simulink model "sampleModel1692"  (R2023a)
settings: Solver=VariableStepAuto  StartTime=0.0  StopTime=10.0  RelTol=1e-3
libraries: hdlsllib x6, simulink x2
settings Model: Creator=user1  LastModifiedBy=user1

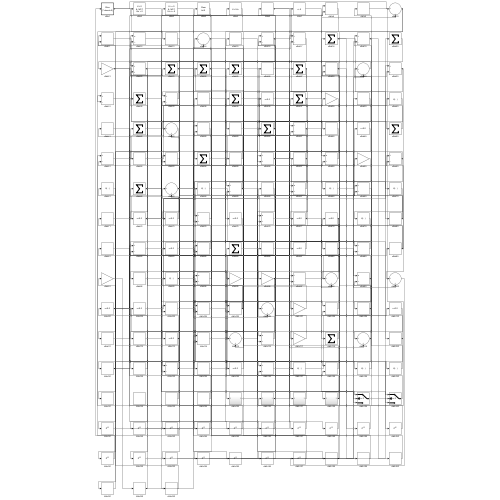
[thumbnail: Simulink's stored preview of the top-level diagram]
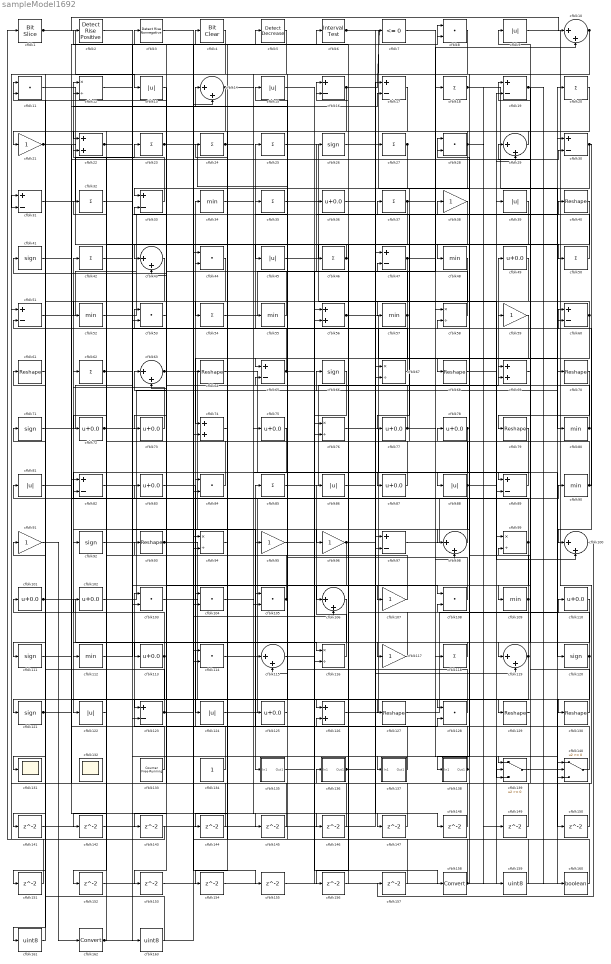
== system sampleModel1692 ==
  cfblk1 : hdlsllib/Logic and Bit Operations/Bit Slice  lidx=7  ridx=0
  cfblk{10,14,29,43,63,98,100,106,115,119} (10 alike) : Sum  Inputs=|++
  cfblk{36,49,72..73,75,77..78,83,87,101..102,110,113,125} (14 alike) : Bias  Bias=0.0  SaturateOnIntegerOverflow=off
  cfblk{8,11,28,44,53,84,103..105,108,114,128} (12 alike) : DotProduct  OutDataTypeStr=Inherit: Inherit via internal rule
  cfblk{21,38,59,91,95..96,107,117} (8 alike) : Gain
  cfblk{34,48,52,55,57,80,90,109,112} (9 alike) : MinMax
  cfblk{26,41,66,71,92,111,120..121} (8 alike) : Signum
  cfblk{12,58,67,76,94,99,116} (7 alike) : Product  Inputs=*/  RndMeth=Zero  SaturateOnIntegerOverflow=on
  cfblk{18,20,23..25,27,32,35,37,42,46,50,54,62,85,118} (16 alike) : Sum  Inputs=+
  cfblk{9,13,15,39,45,81,86,88,122,124} (10 alike) : Abs  SaturateOnIntegerOverflow=off
  cfblk{16..17,19,30..31,33,47,51,60,65,82,89,97,123} (14 alike) : Sum  Inputs=+-
  cfblk{22,56,69,74,126} (5 alike) : Sum
  cfblk{40,61,64,68,70,79,93,127,129..130} (10 alike) : Reshape
  cfblk131 : Scope
  cfblk132 : Scope
      settings: Floating=on
  cfblk133 : hdlsllib/Sources/Counter Free-Running  NumBits=16  tsamp=-1
  cfblk134 : Constant  SampleTime=-1
  cfblk135 : Subsystem
      settings: LibrarySourceBlock=|
      | hdlsllib/Ports &
      | Subsystems/Subsystem
  cfblk136 : Subsystem
      settings: LibrarySourceBlock=|
      | hdlsllib/Ports &
      | Subsystems/Subsystem
  cfblk137 : Subsystem
      settings: LibrarySourceBlock=|
      | hdlsllib/Ports &
      | Subsystems/Subsystem
  cfblk138 : Subsystem
      settings: LibrarySourceBlock=|
      | hdlsllib/Ports &
      | Subsystems/Subsystem
  cfblk139 : Switch  SaturateOnIntegerOverflow=off  InputSameDT=off
  cfblk140 : Switch  SaturateOnIntegerOverflow=off  InputSameDT=off
  cfblk{141..157} (17 alike) : Delay  SampleTime=1
  cfblk158 : DataTypeConversion  SaturateOnIntegerOverflow=off  RndMeth=Floor
  cfblk159 : DataTypeConversion  OutDataTypeStr=uint8  SaturateOnIntegerOverflow=off  RndMeth=Floor
  cfblk160 : DataTypeConversion  OutDataTypeStr=boolean  SaturateOnIntegerOverflow=off  RndMeth=Floor
  cfblk161 : DataTypeConversion  OutDataTypeStr=uint8  SaturateOnIntegerOverflow=off  RndMeth=Floor
  cfblk162 : DataTypeConversion  SaturateOnIntegerOverflow=off  RndMeth=Floor
  cfblk163 : DataTypeConversion  OutDataTypeStr=uint8  SaturateOnIntegerOverflow=off  RndMeth=Floor
  cfblk2 : hdlsllib/Logic and Bit Operations/Detect Rise Positive  vinit=0  OutDataTypeStr=boolean
  cfblk3 : hdlsllib/Logic and Bit Operations/Detect Rise Nonnegative  vinit=0  OutDataTypeStr=boolean
  cfblk4 : simulink/Logic and Bit Operations/Bit Clear  iBit=0
      settings: LibrarySourceBlock=|
      | hdlsllib/Logic and Bit
      | Operations/Bit Clear
  cfblk5 : simulink/Logic and Bit Operations/Detect Decrease  vinit=0.0  OutDataTypeStr=boolean
      settings: LibrarySourceBlock=|
      | hdlsllib/Logic and Bit
      | Operations/Detect
      | Decrease
  cfblk6 : hdlsllib/Logic and Bit Operations/Interval Test  IntervalClosedRight=on  uplimit=0.5  IntervalClosedLeft=on  lowlimit=-0.5  OutDataTypeStr=boolean
  cfblk7 : hdlsllib/Logic and Bit Operations/Compare To Zero  relop=<=  OutDataTypeStr=boolean
  wires:
  cfblk140/1 -> cfblk34/1
  cfblk73/1 -> cfblk42/1
  cfblk55/1 -> cfblk33/1
  cfblk83/1 -> cfblk124/1
  cfblk23/1 -> cfblk65/1, cfblk106/2
  cfblk52/1 -> cfblk38/1
  cfblk44/1 -> cfblk54/1
  cfblk6/1 -> cfblk68/1, cfblk139/3
  cfblk101/1 -> cfblk116/1, cfblk90/1, cfblk8/1
  cfblk85/1 -> cfblk49/1
  cfblk129/1 -> cfblk9/1
  cfblk121/1 -> cfblk61/1, cfblk128/2, cfblk17/2
  cfblk127/1 -> cfblk110/1
  cfblk63/1 -> cfblk135/1(In1), cfblk55/1
  cfblk45/1 -> cfblk48/1
  cfblk77/1 -> cfblk41/1, cfblk139/1
  cfblk79/1 -> cfblk122/1
  cfblk99/1 -> cfblk62/1, cfblk126/1
  cfblk9/1 -> cfblk136/1(In1)
  cfblk98/1 -> cfblk33/2
  cfblk29/1 -> cfblk21/1
  cfblk67/1 -> cfblk25/1
  cfblk118/1 -> cfblk112/1
  cfblk105/1 -> cfblk63/2, cfblk22/2
  cfblk60/1 -> cfblk138/1(In1), cfblk57/1
  cfblk92/1 -> cfblk84/1
  cfblk76/1 -> cfblk89/1
  cfblk48/1 -> cfblk84/2
  cfblk25/1 -> cfblk99/1
  cfblk103/1 -> cfblk129/1
  cfblk69/1 -> cfblk109/1
  cfblk1/1 -> cfblk13/1, cfblk10/1
  cfblk102/1 -> cfblk66/1
  cfblk133/1 -> cfblk103/1
  cfblk7/1 -> cfblk118/1
  cfblk50/1 -> cfblk26/1
  cfblk72/1 -> cfblk44/1, cfblk139/2
  cfblk24/1 -> cfblk88/1, cfblk104/1
  cfblk126/1 -> cfblk60/1
  cfblk113/1 -> cfblk121/1, cfblk101/1
  cfblk41/1 -> cfblk127/1
  cfblk15/1 -> cfblk158/1
  cfblk51/1 -> cfblk14/2
  cfblk31/1 -> cfblk23/1
  cfblk107/1 -> cfblk3/1
  cfblk91/1 -> cfblk162/1
  cfblk117/1 -> cfblk2/1
  cfblk65/1 -> cfblk137/1(In1), cfblk11/2
  cfblk16/1 -> cfblk7/1, cfblk53/2
  cfblk82/1 -> cfblk20/1
  cfblk123/1 -> cfblk71/1, cfblk8/2
  cfblk97/1 -> cfblk39/1
  cfblk70/1 -> cfblk79/1
  cfblk137/1(Out1) -> cfblk85/1
  cfblk108/1 -> cfblk35/1
  cfblk18/1 -> cfblk70/1, cfblk149/1
  cfblk116/1 -> cfblk86/1
  cfblk11/1 -> cfblk58/1
  cfblk46/1 -> cfblk45/1, cfblk156/1
  cfblk35/1 -> cfblk50/1
  cfblk124/1 -> cfblk47/1
  cfblk38/1 -> cfblk106/1
  cfblk80/1 -> cfblk29/1, cfblk53/1
  cfblk17/1 -> cfblk125/1
  cfblk88/1 -> cfblk92/1, cfblk37/1, cfblk100/2
  cfblk34/1 -> cfblk130/1
  cfblk119/1 -> cfblk81/1, cfblk131/1
  cfblk136/1(Out1) -> cfblk69/1, cfblk16/1
  cfblk75/1 -> cfblk113/1
  cfblk40/1 -> cfblk56/2
  cfblk57/1 -> cfblk74/1, cfblk11/1
  cfblk134/1 -> cfblk93/1
  cfblk89/1 -> cfblk87/1
  cfblk27/1 -> cfblk43/1, cfblk115/2
  cfblk110/1 -> cfblk117/1
  cfblk56/1 -> cfblk27/1, cfblk80/1
  cfblk84/1 -> cfblk43/2
  cfblk10/1 -> cfblk98/1, cfblk105/2
  cfblk96/1 -> cfblk59/1, cfblk119/2, cfblk104/2, cfblk143/1
  cfblk58/1 -> cfblk36/1
  cfblk71/1 -> cfblk5/1
  cfblk5/1 -> cfblk31/2
  cfblk74/1 -> cfblk44/2
  cfblk78/1 -> cfblk103/2, cfblk154/1
  cfblk93/1 -> cfblk140/1, cfblk123/1
  cfblk66/1 -> cfblk116/2
  cfblk94/1 -> cfblk24/1
  cfblk111/1 -> cfblk30/2
  cfblk21/1 -> cfblk74/2, cfblk123/2
  cfblk68/1 -> cfblk29/2
  cfblk42/1 -> cfblk94/2
  cfblk114/1 -> cfblk17/1
  cfblk62/1 -> cfblk58/2, cfblk140/2
  cfblk20/1 -> cfblk64/1
  cfblk22/1 -> cfblk95/1, cfblk72/1
  cfblk19/1 -> cfblk119/1, cfblk160/1
  cfblk87/1 -> cfblk32/1
  cfblk138/1(Out1) -> cfblk28/1, cfblk46/1
  cfblk109/1 -> cfblk83/1, cfblk108/2
  cfblk135/1(Out1) -> cfblk76/2
  cfblk2/1 -> cfblk107/1
  cfblk47/1 -> cfblk96/1, cfblk98/2
  cfblk33/1 -> cfblk12/1
  cfblk90/1 -> cfblk60/2, cfblk6/1, cfblk16/2
  cfblk112/1 -> cfblk40/1
  cfblk115/1 -> cfblk47/2
  cfblk54/1 -> cfblk18/1
  cfblk13/1 -> cfblk73/1
  cfblk37/1 -> cfblk105/1, cfblk10/2
  cfblk28/1 -> cfblk22/1, cfblk77/1, cfblk159/1
  cfblk122/1 -> cfblk102/1
  cfblk30/1 -> cfblk67/2, cfblk100/1
  cfblk64/1 -> cfblk120/1
  cfblk125/1 -> cfblk65/2
  cfblk130/1 -> cfblk69/2
  cfblk86/1 -> cfblk108/1
  cfblk120/1 -> cfblk19/1, cfblk140/3
  cfblk8/1 -> cfblk115/1
  cfblk36/1 -> cfblk97/2
  cfblk128/1 -> cfblk12/2
  cfblk61/1 -> cfblk111/1
  cfblk14/1 -> cfblk75/1, cfblk52/1
  cfblk95/1 -> cfblk128/1
  cfblk43/1 -> cfblk141/1
  cfblk141/1 -> cfblk94/1
  cfblk39/1 -> cfblk142/1
  cfblk142/1 -> cfblk97/1
  cfblk143/1 -> cfblk1/1
  cfblk59/1 -> cfblk144/1
  cfblk144/1 -> cfblk82/1
  cfblk81/1 -> cfblk145/1
  cfblk145/1 -> cfblk51/1
  cfblk104/1 -> cfblk146/1
  cfblk146/1 -> cfblk63/1
  cfblk12/1 -> cfblk147/1
  cfblk147/1 -> cfblk76/1
  cfblk26/1 -> cfblk148/1
  cfblk148/1 -> cfblk67/1
  cfblk149/1 -> cfblk28/2
  cfblk139/1 -> cfblk150/1
  cfblk150/1 -> cfblk99/2
  cfblk49/1 -> cfblk151/1
  cfblk151/1 -> cfblk31/1
  cfblk106/1 -> cfblk152/1
  cfblk152/1 -> cfblk30/1
  cfblk53/1 -> cfblk153/1
  cfblk153/1 -> cfblk56/1
  cfblk154/1 -> cfblk19/2
  cfblk3/1 -> cfblk155/1
  cfblk155/1 -> cfblk89/2
  cfblk156/1 -> cfblk126/2
  cfblk100/1 -> cfblk157/1
  cfblk157/1 -> cfblk14/1
  cfblk158/1 -> cfblk114/1, cfblk78/1
  cfblk159/1 -> cfblk15/1
  cfblk160/1 -> cfblk4/1
  cfblk4/1 -> cfblk161/1
  cfblk161/1 -> cfblk51/2
  cfblk162/1 -> cfblk114/2, cfblk82/2
  cfblk32/1 -> cfblk163/1
  cfblk163/1 -> cfblk91/1

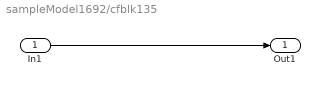
== system sampleModel1692/cfblk135 ==
  In1 : Inport
  Out1 : Outport
  wires:
  In1/1 -> Out1/1

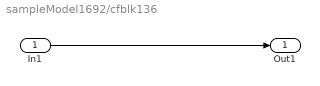
== system sampleModel1692/cfblk136 ==
  In1 : Inport
  Out1 : Outport
  wires:
  In1/1 -> Out1/1

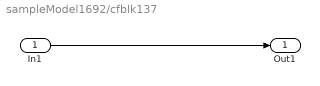
== system sampleModel1692/cfblk137 ==
  In1 : Inport
  Out1 : Outport
  wires:
  In1/1 -> Out1/1

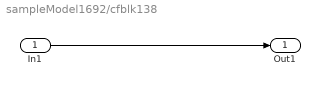
== system sampleModel1692/cfblk138 ==
  In1 : Inport
  Out1 : Outport
  wires:
  In1/1 -> Out1/1
